simulink model "PID"  (R2020a)
settings: Solver=VariableStepAuto  StartTime=0.0  StopTime=10  FixedStep=1/10000  RelTol=1e-3
libraries: cstblocks x2, simulink x1
settings Model: Creator=deniz  LastModifiedBy=deniz

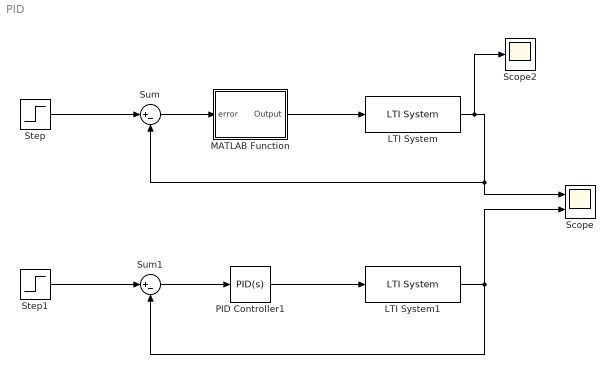
== system PID ==
  LTI System : cstblocks/LTI System  sys=Amp_tf_CW  IC=[]
  LTI System1 : cstblocks/LTI System  sys=Amp_tf_CCW  IC=[]
  MATLAB Function : MATLAB Function  TreatAsAtomicUnit=on
  PID Controller1 : simulink/Continuous/PID Controller  Controller=PID  Form=Parallel  TimeDomain=Continuous-time  UseExternalTs=off  SampleTime=-1  IntegratorMethod=Forward Euler  FilterMethod=Forward Euler  ControllerParametersSource=internal  P=1  I=1  D=1  UseFilter=on  N=5714  TunerSelectOption=Transfer Function Based (PID Tuner App)  InitialConditionSource=internal  InitialConditionForIntegrator=0  InitialConditionForFilter=0  DifferentiatorICPrevScaledInput=0  ExternalReset=none  TrackingMode=off  Kt=1  LimitOutput=off  UpperSaturationLimit=inf  LowerSaturationLimit=-inf  LinearizeAsGain=on  AntiWindupMode=none  Kb=1  POutMin=[]  POutMax=[]  IOutMin=[]  IOutMax=[]  DOutMin=[]  DOutMax=[]  NOutMin=[]  NOutMax=[]  SumOutMin=[]  SumOutMax=[]  SaturationOutMin=[]  SaturationOutMax=[]  PParamMin=[]  PParamMax=[]  IParamMin=[]  IParamMax=[]  DParamMin=[]  DParamMax=[]  NParamMin=[]  NParamMax=[]  KbParamMin=[]  KbParamMax=[]  KtParamMin=[]  KtParamMax=[]  KbOutMin=[]  KbOutMax=[]  KtOutMin=[]  KtOutMax=[]  IntegratorOutMin=[]  IntegratorOutMax=[]  FilterOutMin=[]  FilterOutMax=[]  SumI1OutMin=[]  SumI1OutMax=[]  SumI2OutMin=[]  SumI2OutMax=[]  SumI3OutMin=[]  SumI3OutMax=[]  SumI4OutMin=[]  SumI4OutMax=[]  SumDOutMin=[]  SumDOutMax=[]  DifferentiatorOutMin=[]  DifferentiatorOutMax=[]  FilterDiffOutCoefMin=[]  FilterDiffOutCoefMax=[]  ReciprocalOutMin=[]  ReciprocalOutMax=[]  SumDenOutMin=[]  SumDenOutMax=[]  SumNumOutMin=[]  SumNumOutMax=[]  DivideOutMin=[]  DivideOutMax=[]  UdiffTsProdOutMin=[]  UdiffTsProdOutMax=[]  NTsProdOutMin=[]  NTsProdOutMax=[]  UintegralTsProdOutMin=[]  UintegralTsProdOutMax=[]  UngainTsProdOutMin=[]  UngainTsProdOutMax=[]  IntegratorContinuousStateAttributes=''  IntegratorStateMustResolveToSignalObject=off  IntegratorRTWStateStorageClass=Auto  FilterContinuousStateAttributes=''  FilterStateMustResolveToSignalObject=off  FilterRTWStateStorageClass=Auto  ParallelPVariant=InternalParameters  IdealPVariant=Disabled  IVariant=InternalParameters  DVariant=InternalParameters  IntegratorVariant=Continuous  SatVariant=Disabled  AWVariant=Passthrough  PCopyVariant=Disabled  TRVariant=Disabled  FdbkBlocksVariant=Forward  IdealPFdbkVariant=Disabled  SatFdbkVariant=Disabled  DerivativeFilterVariant=ContFilter  NVariant=InternalParameters  NCopyVariant=Disabled  FilterICVariant=InternalICsFilter  IntegratorICVariant=InternalICs  ExternalResetVariant=Disabled  TRSumVariant=Passthrough  SumFdbkVariant=Disabled  SumVariant=Sum_PID  TsampFilterVariant=InternalTs  TsampNgainVariant=Passthrough  TsampIntegralVariant=Passthrough
  Scope : Scope  NumInputPorts=2
  Scope2 : Scope
  Step : Step  SampleTime=0
  Step1 : Step  SampleTime=0
  Sum : Sum  Inputs=|+-
  Sum1 : Sum  Inputs=|+-
  wires:
  Sum/1 -> MATLAB Function/1(error)
  Step/1 -> Sum/1
  LTI System/1 -> Scope2/1, Sum/2, Scope/1
  PID Controller1/1 -> LTI System1/1
  Step1/1 -> Sum1/1
  Sum1/1 -> PID Controller1/1
  LTI System1/1 -> Scope/2, Sum1/2
  MATLAB Function/1(Output) -> LTI System/1

== matlab function PID/MATLAB Function ==
  settings: updateMethod=DISCRETE  sampleTime=1/10000
  data: error input; Output output
function Output = PID(error)

persistent ept              %holds the exponentials
persistent results          %holds reccorded derivatives
persistent previous_error   %holds input from last execution for derivative calc
persistent integral         %holds the total integral
CF = 10000;                 %ISR frequency
delta_t = 1/CF;             %Will change according to CF, sampling time
size = 8;                   %can change between 5-10
n = 4;                      %Decaying until n*tau, can be 4 or 5
pole = n*CF/size;
P_gain = 3.1;
D_gain = 0.1;
I_gain = 0.1;

%initialize vectors and variables
if isempty(results)
    results = zeros(1,size);
    ept = zeros(1,size);
    sum = 0;
    integral = 0;
    previous_error = 0;
    
    %calculate scale factor for derivative
    for i = 1:size
        sum = sum + pole*exp(-pole*i*delta_t);
    end
    Scale_Factor = 1/(sum);
    
    %properly create ept
    for i = 1:size
        ept(i) = Scale_Factor*pole*exp(-pole*i*delta_t);
    end
end

%Calculating the D(Derivative) of PID
results(2:size)=results(1:size-1);
results(1)=(error - previous_error)/delta_t;
previous_error = error;
derivative = dot(results,ept);

%Calculating the I(Integral) of PID
integral = integral + (error + previous_error)/2*delta_t;

%Calculating the P(Proportional) of PID
proportional = error*P_gain;

Output = proportional + I_gain*integral + D_gain*derivative;
